simulink model "practice1_simulink"  (R2024a)
settings: Solver=ode1  StartTime=0.0  StopTime=10  FixedStep=0.002  RelTol=1e-3  EnableMultiTasking=on
values from neighbouring files (symbols this model uses):
  jeq = jm + jh + jd    (= 1.8351573e-05)    [practice1_script.m]
  km = 0.0422    [practice1_script.m]
  kt = 0.0422    [practice1_script.m]
  rm = 7.5    [practice1_script.m]
undefined symbols (not defined in the file or in its folder): HIL, qc_get_step_size
libraries: quarc_library x6
settings Model: ExtModeTrigDuration=10000  Creator=A00834778  LastModifiedBy=JUAN AUQUILLA
settings SolverCC: AlgebraicLoopSolver=TrustRegion  PositivePriorityOrder=on
settings DataIOCC: ReturnWorkspaceOutputs=off
settings DebuggingCC: UnconnectedInputMsg=warning  UnconnectedOutputMsg=warning  UnconnectedLineMsg=warning  ArithmeticOperatorsInVariantConditions=warning
settings ModelReferenceCC: EnableRefExpFcnMdlSchedulingChecks=on
settings SFSimCC: SimUseLocalCustomCode=off  CustomCodeUndefinedFunction=UseInterfaceOnly
settings RTWCC: Description=QUARC Win64 Target Using Toolchain  SystemTargetFile=quarc_win64.tlc  TemplateMakefile=quarc_default_tmf  RTWUseLocalCustomCode=off  Toolchain=QUARC win64 | nmake (64-bit Windows)  BuildConfiguration=Faster Runs  GPUComputeCapability=3.5
settings CodeAppCC: StateflowObjectComments=on
settings STFCustomTargetCC: ConcurrentExecutionCompliant=on  SystemTargetFile=quarc_win64.tlc
settings GRTTargetCC: ParMdlRefBuildCompliant=off  CompOptLevelCompliant=off  CombineOutputUpdateFcns=off  MatFileLogging=off  CPPClassGenCompliant=off  GRTInterface=on  ExtMode=on  ExtModeMexFile=quarc_comm
settings ConfigComp: CovMetricSettings=dswe

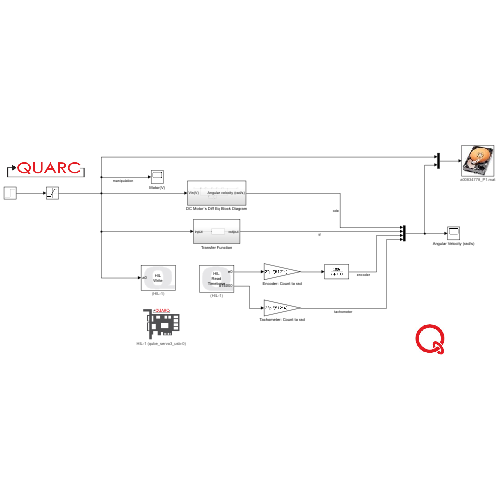
[thumbnail: Simulink's stored preview of the top-level diagram]
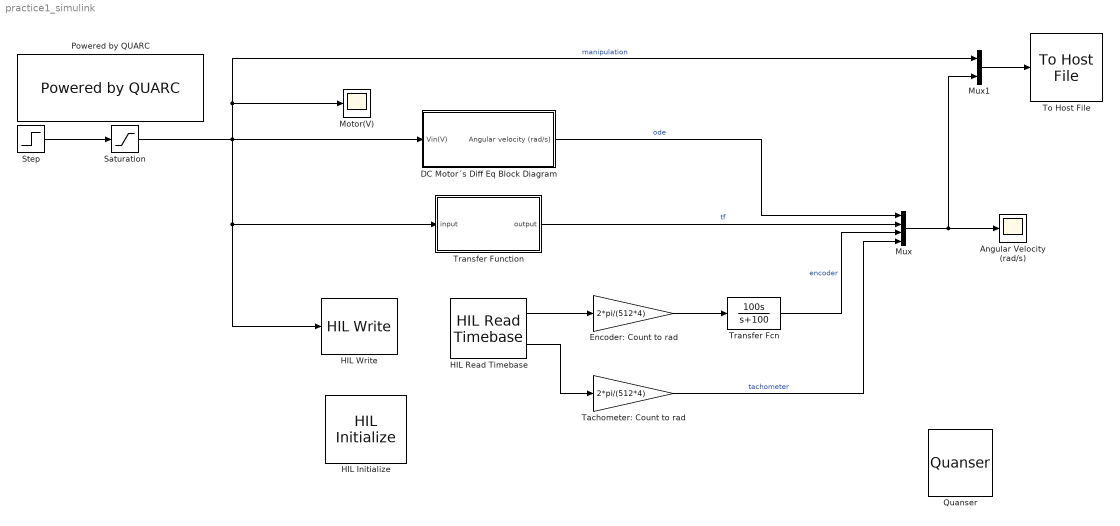
== system practice1_simulink ==
  Angular Velocity (rad/s) : Scope
  DC Motor´s Diff Eq Block Diagram : Subsystem
  Encoder: Count to rad : Gain  Gain=2*pi/(512*4)
  HIL Initialize : quarc_library/Data Acquisition/Generic/Configuration/HIL Initialize  object_name=HIL-1  board_type=qube_servo3_usb  board_number=0  board_options=deadband_compensation=0.65;pwm_en=0;enc0_velocity=3.0;enc1_velocity=3.0;  exclusive=off  active=on  hardware_clocks=[0]  clock_modes=[]  initial_clock_frequencies=[]  set_clock_params_at_start=off  set_clock_params_at_switch_in=off  set_clock_frequencies_at_start=off  set_clock_frequencies_at_switch_in=off  analog_input_channels=[0]  analog_input_configurations=[]  analog_input_maximums=3  analog_input_minimums=-3  set_analog_input_params_at_start=off  set_analog_input_params_at_switch_in=off  analog_output_channels=[0]  analog_output_maximums=15  analog_output_minimums=-15  initial_analog_outputs=[0]  final_analog_outputs=[0]  watchdog_analog_outputs=0  set_analog_output_params_at_start=off  set_analog_output_params_at_switch_in=off  set_analog_outputs_at_start=on  set_analog_outputs_at_switch_in=off  set_analog_outputs_at_terminate=on  set_analog_outputs_at_switch_out=off  set_analog_outputs_on_watchdog=on  digital_input_channels=[]  digital_output_channels=[0]  digital_output_configuration=[]  initial_digital_outputs=[1]  final_digital_outputs=[0]  watchdog_digital_outputs=[0]  set_digital_output_params_at_start=off  set_digital_output_params_at_switch_in=off  set_digital_outputs_at_start=on  set_digital_outputs_at_switch_in=off  set_digital_outputs_at_terminate=on  set_digital_outputs_at_switch_out=off  set_digital_outputs_on_watchdog=on  encoder_channels=[0:1]  quadrature=[4]  encoder_filter_frequency=[]  initial_encoder_counts=[0]  set_encoder_params_at_start=off  set_encoder_params_at_switch_in=off  set_encoder_counts_at_start=on  set_encoder_counts_at_switch_in=off  pwm_channels=[]  pwm_modes=[0]  pwm_frequency=23195  pwm_configuration=[1]  pwm_alignment=[0]  pwm_polarity=[1]  pwm_leading_deadband=[0]  pwm_trailing_deadband=[0]  initial_pwm_outputs=[0]  final_pwm_outputs=[0]  watchdog_pwm_outputs=[]  set_pwm_params_at_start=off  set_pwm_params_at_switch_in=off  set_pwm_outputs_at_start=off  set_pwm_outputs_at_switch_in=off  set_pwm_outputs_at_terminate=off  set_pwm_outputs_at_switch_out=off  set_pwm_outputs_on_watchdog=off  other_output_channels=[11000:11002]  initial_other_outputs=[0 1 0]  final_other_outputs=[1 0 0]  watchdog_other_outputs=[0 0 1]  set_other_outputs_at_start=on  set_other_outputs_at_switch_in=off  set_other_outputs_at_terminate=on  set_other_outputs_at_switch_out=off  set_other_outputs_on_watchdog=on
  HIL Read Timebase : quarc_library/Data Acquisition/Generic/Timebases/HIL Read Timebase  object_name=HIL-1  clock=0  analog_channels=[]  encoder_channels=[0]  digital_channels=[]  other_channels=[14000]  active=on  vector_output=off  data_type_mode=Inherit via back propagation  encoder_data_type=double  digital_data_type=boolean  overflow_mode=Error on overflow  samples_in_buffer=max(ceil(1/qc_get_step_size), 1)
  HIL Write : quarc_library/Data Acquisition/Generic/Immediate I//O/HIL Write  object_name=HIL-1  analog_channels=[0]  pwm_channels=[]  digital_channels=[]  other_channels=[]  sample_time=-1  active=off  vector_input=off
  Motor(V) : Scope
  Mux : Mux
  Mux1 : Mux  Inputs=2
  Powered by QUARC : quarc_library/Logos/Powered by QUARC
  Quanser : quarc_library/Logos/Quanser
  Saturation : Saturate  UpperLimit=10  LowerLimit=-10
  Step : Step  Time=3  Before=3  After=5  SampleTime=0
  Tachometer: Count to rad : Gain  Gain=2*pi/(512*4)
  To Host File : quarc_library/Sinks/To Host/To Host File  file_name=a00834778_P1.mat  variable_name=data  decimation=1  sample_time=-1  file_format=MAT-file v.4  options=No header or footer  append=off  final_file_name=a00834778_P1.mat  bitrate=2000000
  Transfer Fcn : TransferFcn  Numerator=[100 0]  Denominator=[1 100]
  Transfer Function : Subsystem
  wires:
  DC Motor´s Diff Eq Block Diagram/1(Angular velocity (rad/s)) -> Mux/1  "ode"
  Transfer Function/1(output) -> Mux/2  "tf"
  Mux/1 -> Mux1/2, Angular Velocity (rad/s)/1
  HIL Read Timebase/1 -> Encoder: Count to rad/1
  Encoder: Count to rad/1 -> Transfer Fcn/1
  HIL Read Timebase/2 -> Tachometer: Count to rad/1
  Transfer Fcn/1 -> Mux/3  "encoder"
  Tachometer: Count to rad/1 -> Mux/4  "tachometer"
  Step/1 -> Saturation/1
  Saturation/1 -> Mux1/1, Motor(V)/1, DC Motor´s Diff Eq Block Diagram/1(Vin(V)), HIL Write/1, Transfer Function/1(input)  "manipulation"
  Mux1/1 -> To Host File/1

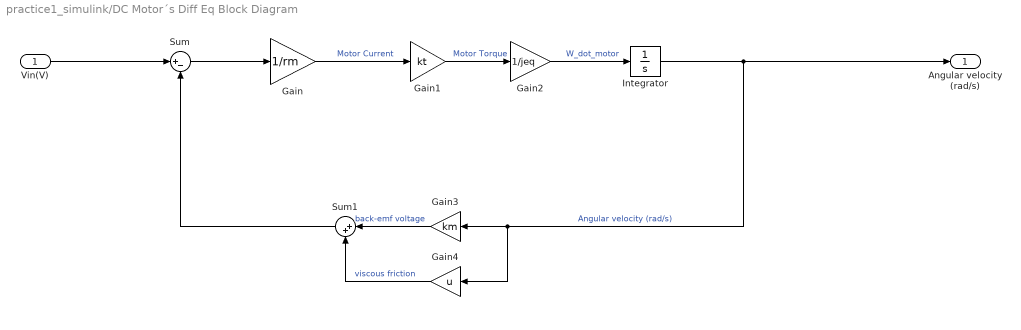
== system practice1_simulink/DC Motor´s Diff Eq Block Diagram ==
  Vin(V) : Inport
  Gain : Gain  Gain=1/rm
  Gain1 : Gain  Gain=kt
  Gain2 : Gain  Gain=1/jeq
  Gain3 : Gain  Gain=km
  Gain4 : Gain  Gain=u
  Integrator : Integrator
  Sum : Sum  Inputs=|+-
  Sum1 : Sum  Inputs=|++
  Angular velocity (rad/s) : Outport
  wires:
  Gain/1 -> Gain1/1  "Motor Current"
  Gain2/1 -> Integrator/1  "W_dot_motor"
  Integrator/1 -> Gain4/1, Gain3/1, Angular velocity (rad/s)/1  "Angular velocity (rad/s)"
  Vin(V)/1 -> Sum/1
  Gain1/1 -> Gain2/1  "Motor Torque"
  Sum/1 -> Gain/1
  Sum1/1 -> Sum/2
  Gain3/1 -> Sum1/1  "back-emf voltage"
  Gain4/1 -> Sum1/2  "viscous friction"

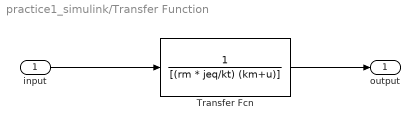
== system practice1_simulink/Transfer Function ==
  input : Inport
  Transfer Fcn : TransferFcn  Denominator=[(rm * jeq/kt) (km+u)]
  output : Outport
  wires:
  input/1 -> Transfer Fcn/1
  Transfer Fcn/1 -> output/1
